simulink model "boat_sim_ss"  (R2018b)
settings: Solver=VariableStepAuto  StartTime=0.0  StopTime=0.1  RelTol=1e-3
values from neighbouring files (symbols this model uses):
  state_eq = ss(eval(real(linearized_A)), eval(real(linearized_B)), C, D)    [ss_linearization.m]
settings Model: Creator=Nicolas  LastModifiedBy=Nicolas

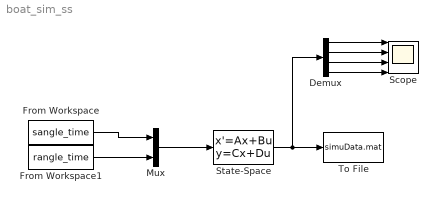
== system boat_sim_ss ==
  Demux : Demux
  From Workspace : FromWorkspace  VariableName=sangle_time  OutDataTypeStr=double  SampleTime=0
  From Workspace1 : FromWorkspace  VariableName=rangle_time  OutDataTypeStr=double  SampleTime=0
  Mux : Mux  Inputs=2
  Scope : Scope  NumInputPorts=4
  State-Space : StateSpace  A=state_eq.a  B=state_eq.b  C=state_eq.c  D=state_eq.d  InitialCondition=0  ContinuousStateAttributes='Velocity'
  To File : ToFile  Filename=simuData.mat  MatrixName=simuData
  wires:
  State-Space/1 -> Demux/1, To File/1
  Mux/1 -> State-Space/1
  From Workspace/1 -> Mux/1
  From Workspace1/1 -> Mux/2
  Demux/1 -> Scope/1
  Demux/2 -> Scope/2
  Demux/3 -> Scope/3
  Demux/4 -> Scope/4
